simulink model "Cruise_control0"  (R2020a)
settings: Solver=VariableStepAuto  StartTime=0.0  StopTime=10.0  RelTol=1e-3
values from neighbouring files (symbols this model uses):
  b = 50.0    [CruiseDD.sldd]
  m = 1000.0    [CruiseDD.sldd]
undefined symbols (not defined in the file or in its folder): Ki, Kp
settings Model: DataDictionary=CruiseDD.sldd  Creator=Admin  LastModifiedBy=Admin
settings DataIOCC: SaveOutput=off  SaveTime=off

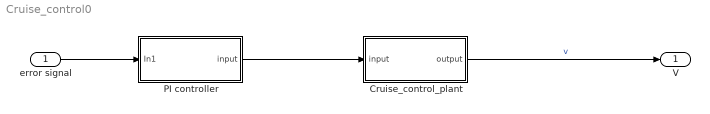
== system Cruise_control0 ==
  error signal : Inport  OutDataTypeStr=double  PortDimensions=1  SampleTime=0
  Cruise_control_plant : Subsystem  TreatAsAtomicUnit=on
  PI controller : Subsystem  TreatAsAtomicUnit=on
  V : Outport  OutDataTypeStr=double  PortDimensions=1  SampleTime=0
  wires:
  PI controller/1(input) -> Cruise_control_plant/1(input)
  Cruise_control_plant/1(output) -> V/1  "v"
  error signal/1 -> PI controller/1(In1)

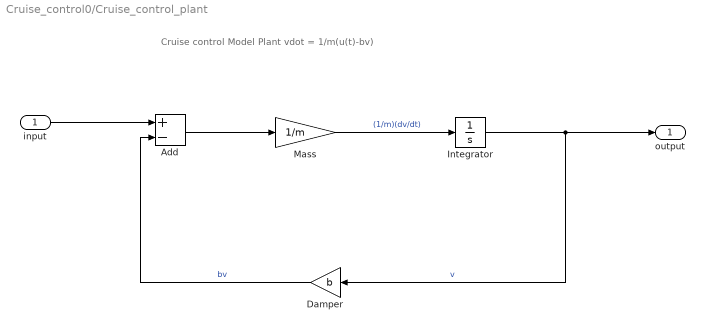
== system Cruise_control0/Cruise_control_plant ==
  note: Cruise control Model Plant
      | vdot = 1/m(u(t)-bv)
  input : Inport
  Add : Sum  Inputs=+-
  Damper : Gain  Gain=b
  Integrator : Integrator
  Mass : Gain  Gain=1/m
  output : Outport
  wires:
  input/1 -> Add/1
  Damper/1 -> Add/2  "bv"
  Add/1 -> Mass/1
  Integrator/1 -> output/1, Damper/1  "v"
  Mass/1 -> Integrator/1  "(1/m)(dv/dt)"

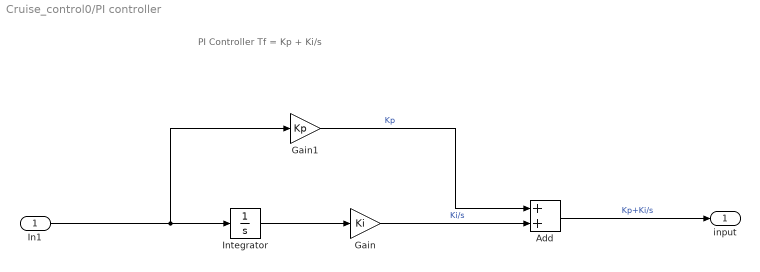
== system Cruise_control0/PI controller ==
  note: PI Controller
      | Tf = Kp + Ki/s
  In1 : Inport
  Add : Sum
  Gain : Gain  Gain=Ki
  Gain1 : Gain  Gain=Kp
  Integrator : Integrator
  input : Outport
  wires:
  Integrator/1 -> Gain/1
  Gain/1 -> Add/2  "Ki/s"
  Add/1 -> input/1  "Kp+Ki/s"
  In1/1 -> Gain1/1, Integrator/1
  Gain1/1 -> Add/1  "Kp"
